simulink subsystem "ReluctanceForceActuator"  (R2025a)
settings: Solver=VariableStepAuto  StartTime=0.0  StopTime=10.0  RelTol=1e-3
model mask{I_max=0, I_min=0, init_airgap=0}
  mask prompts: I_max "Upper Current limit (A):"; I_min "Lower Current limit (A):"; init_airgap "initial air gap (mm)"
libraries: fl_lib x2
settings Model: Creator=Polarstern  LastModifiedBy=CelestialAurora

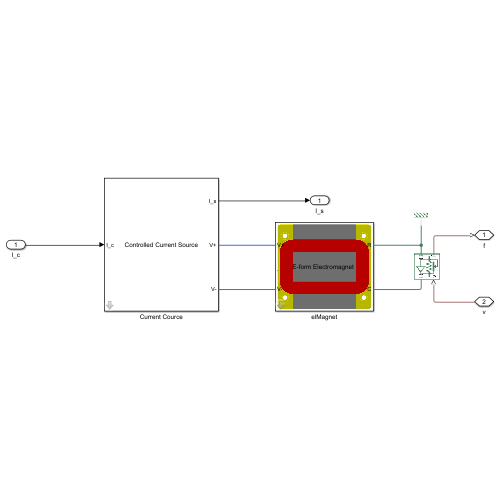
[thumbnail: Simulink's stored preview of the top-level diagram]
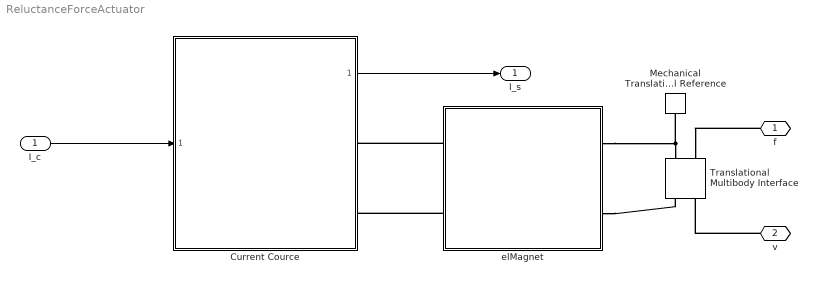
== system ReluctanceForceActuator ==
  I_c : Inport
  Current Cource : Subsystem  ReferencedSubsystem=ControlledCurrentSource  I_max=I_max  I_min=I_min
  Mechanical Translational Reference : fl_lib/Mechanical/Translational Elements/Mechanical Translational Reference
  Translational Multibody Interface : fl_lib/Mechanical/Multibody Interfaces/Translational Multibody Interface
  elMagnet : Subsystem  ReferencedSubsystem=IntegratedElectromagnet  l_airgap=init_airgap
  f : PMIOPort  Side=Left
  v : PMIOPort  Port=2  Side=Right
  I_s : Outport
  wires:
  I_c/1 -> Current Cource/1
  Current Cource/1 -> I_s/1
  connections:
  Translational Multibody Interface/LConn2 -- elMagnet/RConn1 -- Mechanical Translational Reference/LConn1
  elMagnet/LConn2 -- Current Cource/RConn2
  elMagnet/RConn2 -- Translational Multibody Interface/RConn2
  v/RConn1 -- Translational Multibody Interface/RConn1
  elMagnet/LConn1 -- Current Cource/RConn1
  f/RConn1 -- Translational Multibody Interface/LConn1
